simulink model "myBatteryValidationBlockDetailed2RC_IC"  (R2023a)
settings: Solver=daessc  StartTime=0.0  StopTime=1780.8908  MaxStep=1  RelTol=1e-3  AbsTol=1e-3
InitFcn:
  | batteryModelFromBlockDetailed2RC_IC_param
undefined symbols (not defined in the file or in its folder): battery_builder_rtmsupport, gcbh
libraries: batteryModelFromBlockDetailed2RC_IC_lib x36, fl_lib x3, nesl_utility x3
(part 2 of 3)

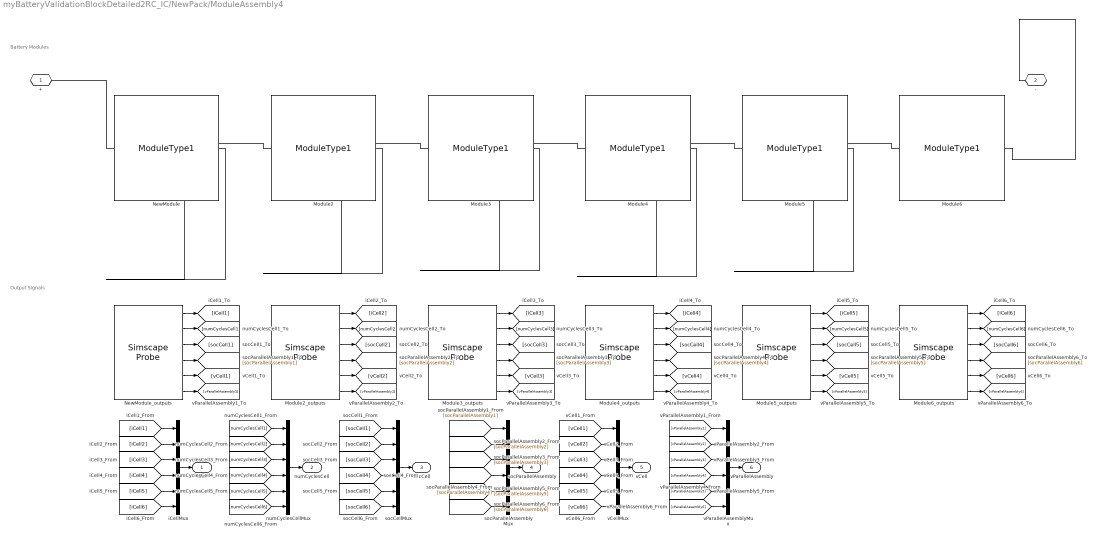
== system myBatteryValidationBlockDetailed2RC_IC/NewPack/ModuleAssembly4 ==
  note: Output Signals
  note: Battery Modules
  Module2 : batteryModelFromBlockDetailed2RC_IC_lib/Modules/ModuleType1  SOC_vecCell=ModuleType1.SOC_vecCell  V0_vecCell=ModuleType1.V0_vecCell V  V_rangeCell=ModuleType1.V_rangeCell V  R0_vecCell=ModuleType1.R0_vecCell Ohm  AHCell=ModuleType1.AHCell A*hr  extrapolation_optionCell=simscape.enum.extrapolation.nearest  R1_vecCell=ModuleType1.R1_vecCell Ohm  tau1_vecCell=ModuleType1.tau1_vecCell s  R2_vecCell=ModuleType1.R2_vecCell Ohm  tau2_vecCell=ModuleType1.tau2_vecCell s  P=1  S=1  iCell_specify=on  iCell_priority=None  iCell=ModuleAssembly4.Module2.iCell A  iCell_nominal_specify=off  iCell_nominal_unit=A  iCell_nominal_value=1  vCell_specify=on  vCell_priority=None  vCell=ModuleAssembly4.Module2.vCell V  vCell_nominal_specify=off  vCell_nominal_unit=V  vCell_nominal_value=1  socCell_specify=on  socCell_priority=High  socCell=ModuleAssembly4.Module2.socCell  socCell_nominal_specify=off  socCell_nominal_unit=1  socCell_nominal_value=1  numCyclesCell_specify=on  numCyclesCell_priority=High  numCyclesCell=ModuleAssembly4.Module2.numCyclesCell  numCyclesCell_nominal_specify=off  numCyclesCell_nominal_unit=1  numCyclesCell_nominal_value=1  vParallelAssembly_specify=on  vParallelAssembly_priority=None  vParallelAssembly=ModuleAssembly4.Module2.vParallelAssembly V  vParallelAssembly_nominal_specify=off  vParallelAssembly_nominal_unit=V  vParallelAssembly_nominal_value=1  socParallelAssembly_specify=on  socParallelAssembly_priority=None  socParallelAssembly=ModuleAssembly4.Module2.socParallelAssembly  socParallelAssembly_nominal_specify=off  socParallelAssembly_nominal_unit=1  socParallelAssembly_nominal_value=1
      settings: InternalSimscapePortConfiguration="{\"Bottom\":[{\"id\":\"n\",\"label\":\"-\",\"type\":\"foundation.electrical.electrical\"}],\"Left\":[],\"Right\":[],\"Top\":[{\"id\":\"p\",\"label\":\"+\",\"type\":\"foundation.electrical.electrical\"}]}"
  Module2_outputs : SimscapeProbe  BoundBlock=3097  Variables={iCell, numCyclesCell, socCell, socParallelAssembly, vCell, vParallelAssembly}
  Module3 : batteryModelFromBlockDetailed2RC_IC_lib/Modules/ModuleType1  SOC_vecCell=ModuleType1.SOC_vecCell  V0_vecCell=ModuleType1.V0_vecCell V  V_rangeCell=ModuleType1.V_rangeCell V  R0_vecCell=ModuleType1.R0_vecCell Ohm  AHCell=ModuleType1.AHCell A*hr  extrapolation_optionCell=simscape.enum.extrapolation.nearest  R1_vecCell=ModuleType1.R1_vecCell Ohm  tau1_vecCell=ModuleType1.tau1_vecCell s  R2_vecCell=ModuleType1.R2_vecCell Ohm  tau2_vecCell=ModuleType1.tau2_vecCell s  P=1  S=1  iCell_specify=on  iCell_priority=None  iCell=ModuleAssembly4.Module3.iCell A  iCell_nominal_specify=off  iCell_nominal_unit=A  iCell_nominal_value=1  vCell_specify=on  vCell_priority=None  vCell=ModuleAssembly4.Module3.vCell V  vCell_nominal_specify=off  vCell_nominal_unit=V  vCell_nominal_value=1  socCell_specify=on  socCell_priority=High  socCell=ModuleAssembly4.Module3.socCell  socCell_nominal_specify=off  socCell_nominal_unit=1  socCell_nominal_value=1  numCyclesCell_specify=on  numCyclesCell_priority=High  numCyclesCell=ModuleAssembly4.Module3.numCyclesCell  numCyclesCell_nominal_specify=off  numCyclesCell_nominal_unit=1  numCyclesCell_nominal_value=1  vParallelAssembly_specify=on  vParallelAssembly_priority=None  vParallelAssembly=ModuleAssembly4.Module3.vParallelAssembly V  vParallelAssembly_nominal_specify=off  vParallelAssembly_nominal_unit=V  vParallelAssembly_nominal_value=1  socParallelAssembly_specify=on  socParallelAssembly_priority=None  socParallelAssembly=ModuleAssembly4.Module3.socParallelAssembly  socParallelAssembly_nominal_specify=off  socParallelAssembly_nominal_unit=1  socParallelAssembly_nominal_value=1
      settings: InternalSimscapePortConfiguration="{\"Bottom\":[{\"id\":\"n\",\"label\":\"-\",\"type\":\"foundation.electrical.electrical\"}],\"Left\":[],\"Right\":[],\"Top\":[{\"id\":\"p\",\"label\":\"+\",\"type\":\"foundation.electrical.electrical\"}]}"
  Module3_outputs : SimscapeProbe  BoundBlock=3099  Variables={iCell, numCyclesCell, socCell, socParallelAssembly, vCell, vParallelAssembly}
  Module4 : batteryModelFromBlockDetailed2RC_IC_lib/Modules/ModuleType1  SOC_vecCell=ModuleType1.SOC_vecCell  V0_vecCell=ModuleType1.V0_vecCell V  V_rangeCell=ModuleType1.V_rangeCell V  R0_vecCell=ModuleType1.R0_vecCell Ohm  AHCell=ModuleType1.AHCell A*hr  extrapolation_optionCell=simscape.enum.extrapolation.nearest  R1_vecCell=ModuleType1.R1_vecCell Ohm  tau1_vecCell=ModuleType1.tau1_vecCell s  R2_vecCell=ModuleType1.R2_vecCell Ohm  tau2_vecCell=ModuleType1.tau2_vecCell s  P=1  S=1  iCell_specify=on  iCell_priority=None  iCell=ModuleAssembly4.Module4.iCell A  iCell_nominal_specify=off  iCell_nominal_unit=A  iCell_nominal_value=1  vCell_specify=on  vCell_priority=None  vCell=ModuleAssembly4.Module4.vCell V  vCell_nominal_specify=off  vCell_nominal_unit=V  vCell_nominal_value=1  socCell_specify=on  socCell_priority=High  socCell=ModuleAssembly4.Module4.socCell  socCell_nominal_specify=off  socCell_nominal_unit=1  socCell_nominal_value=1  numCyclesCell_specify=on  numCyclesCell_priority=High  numCyclesCell=ModuleAssembly4.Module4.numCyclesCell  numCyclesCell_nominal_specify=off  numCyclesCell_nominal_unit=1  numCyclesCell_nominal_value=1  vParallelAssembly_specify=on  vParallelAssembly_priority=None  vParallelAssembly=ModuleAssembly4.Module4.vParallelAssembly V  vParallelAssembly_nominal_specify=off  vParallelAssembly_nominal_unit=V  vParallelAssembly_nominal_value=1  socParallelAssembly_specify=on  socParallelAssembly_priority=None  socParallelAssembly=ModuleAssembly4.Module4.socParallelAssembly  socParallelAssembly_nominal_specify=off  socParallelAssembly_nominal_unit=1  socParallelAssembly_nominal_value=1
      settings: InternalSimscapePortConfiguration="{\"Bottom\":[{\"id\":\"n\",\"label\":\"-\",\"type\":\"foundation.electrical.electrical\"}],\"Left\":[],\"Right\":[],\"Top\":[{\"id\":\"p\",\"label\":\"+\",\"type\":\"foundation.electrical.electrical\"}]}"
  Module4_outputs : SimscapeProbe  BoundBlock=3101  Variables={iCell, numCyclesCell, socCell, socParallelAssembly, vCell, vParallelAssembly}
  Module5 : batteryModelFromBlockDetailed2RC_IC_lib/Modules/ModuleType1  SOC_vecCell=ModuleType1.SOC_vecCell  V0_vecCell=ModuleType1.V0_vecCell V  V_rangeCell=ModuleType1.V_rangeCell V  R0_vecCell=ModuleType1.R0_vecCell Ohm  AHCell=ModuleType1.AHCell A*hr  extrapolation_optionCell=simscape.enum.extrapolation.nearest  R1_vecCell=ModuleType1.R1_vecCell Ohm  tau1_vecCell=ModuleType1.tau1_vecCell s  R2_vecCell=ModuleType1.R2_vecCell Ohm  tau2_vecCell=ModuleType1.tau2_vecCell s  P=1  S=1  iCell_specify=on  iCell_priority=None  iCell=ModuleAssembly4.Module5.iCell A  iCell_nominal_specify=off  iCell_nominal_unit=A  iCell_nominal_value=1  vCell_specify=on  vCell_priority=None  vCell=ModuleAssembly4.Module5.vCell V  vCell_nominal_specify=off  vCell_nominal_unit=V  vCell_nominal_value=1  socCell_specify=on  socCell_priority=High  socCell=ModuleAssembly4.Module5.socCell  socCell_nominal_specify=off  socCell_nominal_unit=1  socCell_nominal_value=1  numCyclesCell_specify=on  numCyclesCell_priority=High  numCyclesCell=ModuleAssembly4.Module5.numCyclesCell  numCyclesCell_nominal_specify=off  numCyclesCell_nominal_unit=1  numCyclesCell_nominal_value=1  vParallelAssembly_specify=on  vParallelAssembly_priority=None  vParallelAssembly=ModuleAssembly4.Module5.vParallelAssembly V  vParallelAssembly_nominal_specify=off  vParallelAssembly_nominal_unit=V  vParallelAssembly_nominal_value=1  socParallelAssembly_specify=on  socParallelAssembly_priority=None  socParallelAssembly=ModuleAssembly4.Module5.socParallelAssembly  socParallelAssembly_nominal_specify=off  socParallelAssembly_nominal_unit=1  socParallelAssembly_nominal_value=1
      settings: InternalSimscapePortConfiguration="{\"Bottom\":[{\"id\":\"n\",\"label\":\"-\",\"type\":\"foundation.electrical.electrical\"}],\"Left\":[],\"Right\":[],\"Top\":[{\"id\":\"p\",\"label\":\"+\",\"type\":\"foundation.electrical.electrical\"}]}"
  Module5_outputs : SimscapeProbe  BoundBlock=3103  Variables={iCell, numCyclesCell, socCell, socParallelAssembly, vCell, vParallelAssembly}
  Module6 : batteryModelFromBlockDetailed2RC_IC_lib/Modules/ModuleType1  SOC_vecCell=ModuleType1.SOC_vecCell  V0_vecCell=ModuleType1.V0_vecCell V  V_rangeCell=ModuleType1.V_rangeCell V  R0_vecCell=ModuleType1.R0_vecCell Ohm  AHCell=ModuleType1.AHCell A*hr  extrapolation_optionCell=simscape.enum.extrapolation.nearest  R1_vecCell=ModuleType1.R1_vecCell Ohm  tau1_vecCell=ModuleType1.tau1_vecCell s  R2_vecCell=ModuleType1.R2_vecCell Ohm  tau2_vecCell=ModuleType1.tau2_vecCell s  P=1  S=1  iCell_specify=on  iCell_priority=None  iCell=ModuleAssembly4.Module6.iCell A  iCell_nominal_specify=off  iCell_nominal_unit=A  iCell_nominal_value=1  vCell_specify=on  vCell_priority=None  vCell=ModuleAssembly4.Module6.vCell V  vCell_nominal_specify=off  vCell_nominal_unit=V  vCell_nominal_value=1  socCell_specify=on  socCell_priority=High  socCell=ModuleAssembly4.Module6.socCell  socCell_nominal_specify=off  socCell_nominal_unit=1  socCell_nominal_value=1  numCyclesCell_specify=on  numCyclesCell_priority=High  numCyclesCell=ModuleAssembly4.Module6.numCyclesCell  numCyclesCell_nominal_specify=off  numCyclesCell_nominal_unit=1  numCyclesCell_nominal_value=1  vParallelAssembly_specify=on  vParallelAssembly_priority=None  vParallelAssembly=ModuleAssembly4.Module6.vParallelAssembly V  vParallelAssembly_nominal_specify=off  vParallelAssembly_nominal_unit=V  vParallelAssembly_nominal_value=1  socParallelAssembly_specify=on  socParallelAssembly_priority=None  socParallelAssembly=ModuleAssembly4.Module6.socParallelAssembly  socParallelAssembly_nominal_specify=off  socParallelAssembly_nominal_unit=1  socParallelAssembly_nominal_value=1
      settings: InternalSimscapePortConfiguration="{\"Bottom\":[{\"id\":\"n\",\"label\":\"-\",\"type\":\"foundation.electrical.electrical\"}],\"Left\":[],\"Right\":[],\"Top\":[{\"id\":\"p\",\"label\":\"+\",\"type\":\"foundation.electrical.electrical\"}]}"
  Module6_outputs : SimscapeProbe  BoundBlock=3105  Variables={iCell, numCyclesCell, socCell, socParallelAssembly, vCell, vParallelAssembly}
  NewModule : batteryModelFromBlockDetailed2RC_IC_lib/Modules/ModuleType1  SOC_vecCell=ModuleType1.SOC_vecCell  V0_vecCell=ModuleType1.V0_vecCell V  V_rangeCell=ModuleType1.V_rangeCell V  R0_vecCell=ModuleType1.R0_vecCell Ohm  AHCell=ModuleType1.AHCell A*hr  extrapolation_optionCell=simscape.enum.extrapolation.nearest  R1_vecCell=ModuleType1.R1_vecCell Ohm  tau1_vecCell=ModuleType1.tau1_vecCell s  R2_vecCell=ModuleType1.R2_vecCell Ohm  tau2_vecCell=ModuleType1.tau2_vecCell s  P=1  S=1  iCell_specify=on  iCell_priority=None  iCell=ModuleAssembly4.NewModule.iCell A  iCell_nominal_specify=off  iCell_nominal_unit=A  iCell_nominal_value=1  vCell_specify=on  vCell_priority=None  vCell=ModuleAssembly4.NewModule.vCell V  vCell_nominal_specify=off  vCell_nominal_unit=V  vCell_nominal_value=1  socCell_specify=on  socCell_priority=High  socCell=ModuleAssembly4.NewModule.socCell  socCell_nominal_specify=off  socCell_nominal_unit=1  socCell_nominal_value=1  numCyclesCell_specify=on  numCyclesCell_priority=High  numCyclesCell=ModuleAssembly4.NewModule.numCyclesCell  numCyclesCell_nominal_specify=off  numCyclesCell_nominal_unit=1  numCyclesCell_nominal_value=1  vParallelAssembly_specify=on  vParallelAssembly_priority=None  vParallelAssembly=ModuleAssembly4.NewModule.vParallelAssembly V  vParallelAssembly_nominal_specify=off  vParallelAssembly_nominal_unit=V  vParallelAssembly_nominal_value=1  socParallelAssembly_specify=on  socParallelAssembly_priority=None  socParallelAssembly=ModuleAssembly4.NewModule.socParallelAssembly  socParallelAssembly_nominal_specify=off  socParallelAssembly_nominal_unit=1  socParallelAssembly_nominal_value=1
      settings: InternalSimscapePortConfiguration="{\"Bottom\":[{\"id\":\"n\",\"label\":\"-\",\"type\":\"foundation.electrical.electrical\"}],\"Left\":[],\"Right\":[],\"Top\":[{\"id\":\"p\",\"label\":\"+\",\"type\":\"foundation.electrical.electrical\"}]}"
  NewModule_outputs : SimscapeProbe  BoundBlock=3107  Variables={iCell, numCyclesCell, socCell, socParallelAssembly, vCell, vParallelAssembly}
  iCellMux : Mux  Inputs=6
  numCyclesCellMux : Mux  Inputs=6
  socCellMux : Mux  Inputs=6
  socParallelAssemblyMux : Mux  Inputs=6
  vCellMux : Mux  Inputs=6
  vParallelAssemblyMux : Mux  Inputs=6
  + : PMIOPort  Side=Left
  - : PMIOPort  Port=2  Side=Right
  iCell : Outport
  numCyclesCell : Outport  Port=2
  socCell : Outport  Port=3
  socParallelAssembly : Outport  Port=4
  vCell : Outport  Port=5
  vParallelAssembly : Outport  Port=6
  wires:
  [vParallelAssembly6] -> vParallelAssemblyMux/6
  Module6_outputs/6 -> [vParallelAssembly6]
  [vCell6] -> vCellMux/6
  Module6_outputs/5 -> [vCell6]
  [socParallelAssembly6] -> socParallelAssemblyMux/6
  Module6_outputs/4 -> [socParallelAssembly6]
  [socCell6] -> socCellMux/6
  Module6_outputs/3 -> [socCell6]
  [numCyclesCell6] -> numCyclesCellMux/6
  Module6_outputs/2 -> [numCyclesCell6]
  [iCell6] -> iCellMux/6
  Module6_outputs/1 -> [iCell6]
  [vParallelAssembly5] -> vParallelAssemblyMux/5
  Module5_outputs/6 -> [vParallelAssembly5]
  [vCell5] -> vCellMux/5
  Module5_outputs/5 -> [vCell5]
  [socParallelAssembly5] -> socParallelAssemblyMux/5
  Module5_outputs/4 -> [socParallelAssembly5]
  [socCell5] -> socCellMux/5
  Module5_outputs/3 -> [socCell5]
  [numCyclesCell5] -> numCyclesCellMux/5
  Module5_outputs/2 -> [numCyclesCell5]
  [iCell5] -> iCellMux/5
  Module5_outputs/1 -> [iCell5]
  [vParallelAssembly4] -> vParallelAssemblyMux/4
  Module4_outputs/6 -> [vParallelAssembly4]
  [vCell4] -> vCellMux/4
  Module4_outputs/5 -> [vCell4]
  [socParallelAssembly4] -> socParallelAssemblyMux/4
  Module4_outputs/4 -> [socParallelAssembly4]
  [socCell4] -> socCellMux/4
  Module4_outputs/3 -> [socCell4]
  [numCyclesCell4] -> numCyclesCellMux/4
  Module4_outputs/2 -> [numCyclesCell4]
  [iCell4] -> iCellMux/4
  Module4_outputs/1 -> [iCell4]
  [vParallelAssembly3] -> vParallelAssemblyMux/3
  Module3_outputs/6 -> [vParallelAssembly3]
  [vCell3] -> vCellMux/3
  Module3_outputs/5 -> [vCell3]
  [socParallelAssembly3] -> socParallelAssemblyMux/3
  Module3_outputs/4 -> [socParallelAssembly3]
  [socCell3] -> socCellMux/3
  Module3_outputs/3 -> [socCell3]
  [numCyclesCell3] -> numCyclesCellMux/3
  Module3_outputs/2 -> [numCyclesCell3]
  [iCell3] -> iCellMux/3
  Module3_outputs/1 -> [iCell3]
  [vParallelAssembly2] -> vParallelAssemblyMux/2
  Module2_outputs/6 -> [vParallelAssembly2]
  [vCell2] -> vCellMux/2
  Module2_outputs/5 -> [vCell2]
  [socParallelAssembly2] -> socParallelAssemblyMux/2
  Module2_outputs/4 -> [socParallelAssembly2]
  [socCell2] -> socCellMux/2
  Module2_outputs/3 -> [socCell2]
  [numCyclesCell2] -> numCyclesCellMux/2
  Module2_outputs/2 -> [numCyclesCell2]
  [iCell2] -> iCellMux/2
  Module2_outputs/1 -> [iCell2]
  [vParallelAssembly1] -> vParallelAssemblyMux/1
  vParallelAssemblyMux/1 -> vParallelAssembly/1
  NewModule_outputs/6 -> [vParallelAssembly1]
  [vCell1] -> vCellMux/1
  vCellMux/1 -> vCell/1
  NewModule_outputs/5 -> [vCell1]
  [socParallelAssembly1] -> socParallelAssemblyMux/1
  socParallelAssemblyMux/1 -> socParallelAssembly/1
  NewModule_outputs/4 -> [socParallelAssembly1]
  [socCell1] -> socCellMux/1
  socCellMux/1 -> socCell/1
  NewModule_outputs/3 -> [socCell1]
  [numCyclesCell1] -> numCyclesCellMux/1
  numCyclesCellMux/1 -> numCyclesCell/1
  NewModule_outputs/2 -> [numCyclesCell1]
  [iCell1] -> iCellMux/1
  iCellMux/1 -> iCell/1
  NewModule_outputs/1 -> [iCell1]
  connections:
  Module6/RConn1 -- -/RConn1
  NewModule/LConn1 -- +/RConn1
  Module6/LConn1 -- Module5/RConn1
  Module5/LConn1 -- Module4/RConn1
  Module4/LConn1 -- Module3/RConn1
  Module3/LConn1 -- Module2/RConn1
  Module2/LConn1 -- NewModule/RConn1

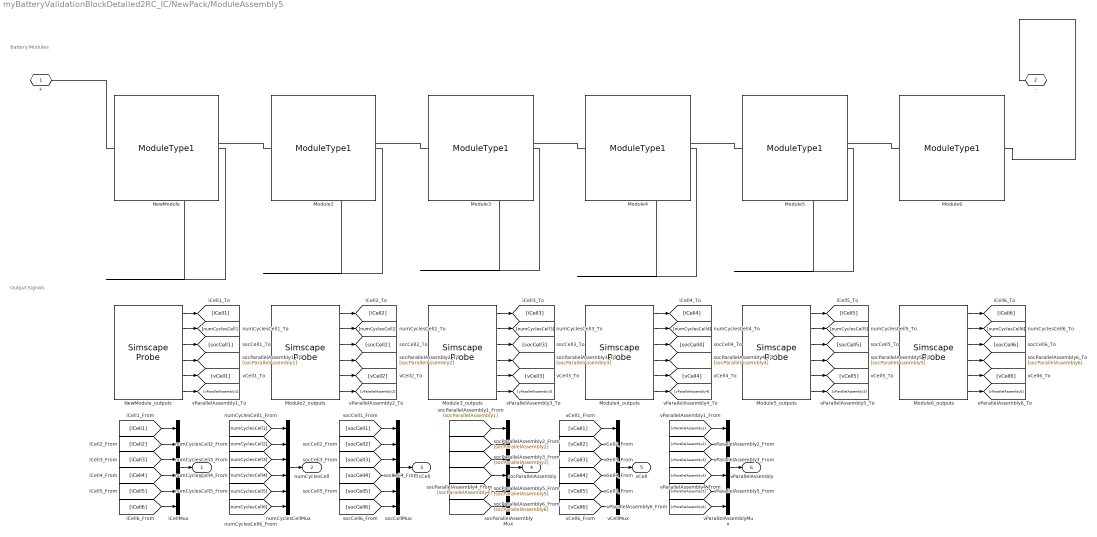
== system myBatteryValidationBlockDetailed2RC_IC/NewPack/ModuleAssembly5 ==
  note: Output Signals
  note: Battery Modules
  Module2 : batteryModelFromBlockDetailed2RC_IC_lib/Modules/ModuleType1  SOC_vecCell=ModuleType1.SOC_vecCell  V0_vecCell=ModuleType1.V0_vecCell V  V_rangeCell=ModuleType1.V_rangeCell V  R0_vecCell=ModuleType1.R0_vecCell Ohm  AHCell=ModuleType1.AHCell A*hr  extrapolation_optionCell=simscape.enum.extrapolation.nearest  R1_vecCell=ModuleType1.R1_vecCell Ohm  tau1_vecCell=ModuleType1.tau1_vecCell s  R2_vecCell=ModuleType1.R2_vecCell Ohm  tau2_vecCell=ModuleType1.tau2_vecCell s  P=1  S=1  iCell_specify=on  iCell_priority=None  iCell=ModuleAssembly5.Module2.iCell A  iCell_nominal_specify=off  iCell_nominal_unit=A  iCell_nominal_value=1  vCell_specify=on  vCell_priority=None  vCell=ModuleAssembly5.Module2.vCell V  vCell_nominal_specify=off  vCell_nominal_unit=V  vCell_nominal_value=1  socCell_specify=on  socCell_priority=High  socCell=ModuleAssembly5.Module2.socCell  socCell_nominal_specify=off  socCell_nominal_unit=1  socCell_nominal_value=1  numCyclesCell_specify=on  numCyclesCell_priority=High  numCyclesCell=ModuleAssembly5.Module2.numCyclesCell  numCyclesCell_nominal_specify=off  numCyclesCell_nominal_unit=1  numCyclesCell_nominal_value=1  vParallelAssembly_specify=on  vParallelAssembly_priority=None  vParallelAssembly=ModuleAssembly5.Module2.vParallelAssembly V  vParallelAssembly_nominal_specify=off  vParallelAssembly_nominal_unit=V  vParallelAssembly_nominal_value=1  socParallelAssembly_specify=on  socParallelAssembly_priority=None  socParallelAssembly=ModuleAssembly5.Module2.socParallelAssembly  socParallelAssembly_nominal_specify=off  socParallelAssembly_nominal_unit=1  socParallelAssembly_nominal_value=1
      settings: InternalSimscapePortConfiguration="{\"Bottom\":[{\"id\":\"n\",\"label\":\"-\",\"type\":\"foundation.electrical.electrical\"}],\"Left\":[],\"Right\":[],\"Top\":[{\"id\":\"p\",\"label\":\"+\",\"type\":\"foundation.electrical.electrical\"}]}"
  Module2_outputs : SimscapeProbe  BoundBlock=3198  Variables={iCell, numCyclesCell, socCell, socParallelAssembly, vCell, vParallelAssembly}
  Module3 : batteryModelFromBlockDetailed2RC_IC_lib/Modules/ModuleType1  SOC_vecCell=ModuleType1.SOC_vecCell  V0_vecCell=ModuleType1.V0_vecCell V  V_rangeCell=ModuleType1.V_rangeCell V  R0_vecCell=ModuleType1.R0_vecCell Ohm  AHCell=ModuleType1.AHCell A*hr  extrapolation_optionCell=simscape.enum.extrapolation.nearest  R1_vecCell=ModuleType1.R1_vecCell Ohm  tau1_vecCell=ModuleType1.tau1_vecCell s  R2_vecCell=ModuleType1.R2_vecCell Ohm  tau2_vecCell=ModuleType1.tau2_vecCell s  P=1  S=1  iCell_specify=on  iCell_priority=None  iCell=ModuleAssembly5.Module3.iCell A  iCell_nominal_specify=off  iCell_nominal_unit=A  iCell_nominal_value=1  vCell_specify=on  vCell_priority=None  vCell=ModuleAssembly5.Module3.vCell V  vCell_nominal_specify=off  vCell_nominal_unit=V  vCell_nominal_value=1  socCell_specify=on  socCell_priority=High  socCell=ModuleAssembly5.Module3.socCell  socCell_nominal_specify=off  socCell_nominal_unit=1  socCell_nominal_value=1  numCyclesCell_specify=on  numCyclesCell_priority=High  numCyclesCell=ModuleAssembly5.Module3.numCyclesCell  numCyclesCell_nominal_specify=off  numCyclesCell_nominal_unit=1  numCyclesCell_nominal_value=1  vParallelAssembly_specify=on  vParallelAssembly_priority=None  vParallelAssembly=ModuleAssembly5.Module3.vParallelAssembly V  vParallelAssembly_nominal_specify=off  vParallelAssembly_nominal_unit=V  vParallelAssembly_nominal_value=1  socParallelAssembly_specify=on  socParallelAssembly_priority=None  socParallelAssembly=ModuleAssembly5.Module3.socParallelAssembly  socParallelAssembly_nominal_specify=off  socParallelAssembly_nominal_unit=1  socParallelAssembly_nominal_value=1
      settings: InternalSimscapePortConfiguration="{\"Bottom\":[{\"id\":\"n\",\"label\":\"-\",\"type\":\"foundation.electrical.electrical\"}],\"Left\":[],\"Right\":[],\"Top\":[{\"id\":\"p\",\"label\":\"+\",\"type\":\"foundation.electrical.electrical\"}]}"
  Module3_outputs : SimscapeProbe  BoundBlock=3200  Variables={iCell, numCyclesCell, socCell, socParallelAssembly, vCell, vParallelAssembly}
  Module4 : batteryModelFromBlockDetailed2RC_IC_lib/Modules/ModuleType1  SOC_vecCell=ModuleType1.SOC_vecCell  V0_vecCell=ModuleType1.V0_vecCell V  V_rangeCell=ModuleType1.V_rangeCell V  R0_vecCell=ModuleType1.R0_vecCell Ohm  AHCell=ModuleType1.AHCell A*hr  extrapolation_optionCell=simscape.enum.extrapolation.nearest  R1_vecCell=ModuleType1.R1_vecCell Ohm  tau1_vecCell=ModuleType1.tau1_vecCell s  R2_vecCell=ModuleType1.R2_vecCell Ohm  tau2_vecCell=ModuleType1.tau2_vecCell s  P=1  S=1  iCell_specify=on  iCell_priority=None  iCell=ModuleAssembly5.Module4.iCell A  iCell_nominal_specify=off  iCell_nominal_unit=A  iCell_nominal_value=1  vCell_specify=on  vCell_priority=None  vCell=ModuleAssembly5.Module4.vCell V  vCell_nominal_specify=off  vCell_nominal_unit=V  vCell_nominal_value=1  socCell_specify=on  socCell_priority=High  socCell=ModuleAssembly5.Module4.socCell  socCell_nominal_specify=off  socCell_nominal_unit=1  socCell_nominal_value=1  numCyclesCell_specify=on  numCyclesCell_priority=High  numCyclesCell=ModuleAssembly5.Module4.numCyclesCell  numCyclesCell_nominal_specify=off  numCyclesCell_nominal_unit=1  numCyclesCell_nominal_value=1  vParallelAssembly_specify=on  vParallelAssembly_priority=None  vParallelAssembly=ModuleAssembly5.Module4.vParallelAssembly V  vParallelAssembly_nominal_specify=off  vParallelAssembly_nominal_unit=V  vParallelAssembly_nominal_value=1  socParallelAssembly_specify=on  socParallelAssembly_priority=None  socParallelAssembly=ModuleAssembly5.Module4.socParallelAssembly  socParallelAssembly_nominal_specify=off  socParallelAssembly_nominal_unit=1  socParallelAssembly_nominal_value=1
      settings: InternalSimscapePortConfiguration="{\"Bottom\":[{\"id\":\"n\",\"label\":\"-\",\"type\":\"foundation.electrical.electrical\"}],\"Left\":[],\"Right\":[],\"Top\":[{\"id\":\"p\",\"label\":\"+\",\"type\":\"foundation.electrical.electrical\"}]}"
  Module4_outputs : SimscapeProbe  BoundBlock=3202  Variables={iCell, numCyclesCell, socCell, socParallelAssembly, vCell, vParallelAssembly}
  Module5 : batteryModelFromBlockDetailed2RC_IC_lib/Modules/ModuleType1  SOC_vecCell=ModuleType1.SOC_vecCell  V0_vecCell=ModuleType1.V0_vecCell V  V_rangeCell=ModuleType1.V_rangeCell V  R0_vecCell=ModuleType1.R0_vecCell Ohm  AHCell=ModuleType1.AHCell A*hr  extrapolation_optionCell=simscape.enum.extrapolation.nearest  R1_vecCell=ModuleType1.R1_vecCell Ohm  tau1_vecCell=ModuleType1.tau1_vecCell s  R2_vecCell=ModuleType1.R2_vecCell Ohm  tau2_vecCell=ModuleType1.tau2_vecCell s  P=1  S=1  iCell_specify=on  iCell_priority=None  iCell=ModuleAssembly5.Module5.iCell A  iCell_nominal_specify=off  iCell_nominal_unit=A  iCell_nominal_value=1  vCell_specify=on  vCell_priority=None  vCell=ModuleAssembly5.Module5.vCell V  vCell_nominal_specify=off  vCell_nominal_unit=V  vCell_nominal_value=1  socCell_specify=on  socCell_priority=High  socCell=ModuleAssembly5.Module5.socCell  socCell_nominal_specify=off  socCell_nominal_unit=1  socCell_nominal_value=1  numCyclesCell_specify=on  numCyclesCell_priority=High  numCyclesCell=ModuleAssembly5.Module5.numCyclesCell  numCyclesCell_nominal_specify=off  numCyclesCell_nominal_unit=1  numCyclesCell_nominal_value=1  vParallelAssembly_specify=on  vParallelAssembly_priority=None  vParallelAssembly=ModuleAssembly5.Module5.vParallelAssembly V  vParallelAssembly_nominal_specify=off  vParallelAssembly_nominal_unit=V  vParallelAssembly_nominal_value=1  socParallelAssembly_specify=on  socParallelAssembly_priority=None  socParallelAssembly=ModuleAssembly5.Module5.socParallelAssembly  socParallelAssembly_nominal_specify=off  socParallelAssembly_nominal_unit=1  socParallelAssembly_nominal_value=1
      settings: InternalSimscapePortConfiguration="{\"Bottom\":[{\"id\":\"n\",\"label\":\"-\",\"type\":\"foundation.electrical.electrical\"}],\"Left\":[],\"Right\":[],\"Top\":[{\"id\":\"p\",\"label\":\"+\",\"type\":\"foundation.electrical.electrical\"}]}"
  Module5_outputs : SimscapeProbe  BoundBlock=3204  Variables={iCell, numCyclesCell, socCell, socParallelAssembly, vCell, vParallelAssembly}
  Module6 : batteryModelFromBlockDetailed2RC_IC_lib/Modules/ModuleType1  SOC_vecCell=ModuleType1.SOC_vecCell  V0_vecCell=ModuleType1.V0_vecCell V  V_rangeCell=ModuleType1.V_rangeCell V  R0_vecCell=ModuleType1.R0_vecCell Ohm  AHCell=ModuleType1.AHCell A*hr  extrapolation_optionCell=simscape.enum.extrapolation.nearest  R1_vecCell=ModuleType1.R1_vecCell Ohm  tau1_vecCell=ModuleType1.tau1_vecCell s  R2_vecCell=ModuleType1.R2_vecCell Ohm  tau2_vecCell=ModuleType1.tau2_vecCell s  P=1  S=1  iCell_specify=on  iCell_priority=None  iCell=ModuleAssembly5.Module6.iCell A  iCell_nominal_specify=off  iCell_nominal_unit=A  iCell_nominal_value=1  vCell_specify=on  vCell_priority=None  vCell=ModuleAssembly5.Module6.vCell V  vCell_nominal_specify=off  vCell_nominal_unit=V  vCell_nominal_value=1  socCell_specify=on  socCell_priority=High  socCell=ModuleAssembly5.Module6.socCell  socCell_nominal_specify=off  socCell_nominal_unit=1  socCell_nominal_value=1  numCyclesCell_specify=on  numCyclesCell_priority=High  numCyclesCell=ModuleAssembly5.Module6.numCyclesCell  numCyclesCell_nominal_specify=off  numCyclesCell_nominal_unit=1  numCyclesCell_nominal_value=1  vParallelAssembly_specify=on  vParallelAssembly_priority=None  vParallelAssembly=ModuleAssembly5.Module6.vParallelAssembly V  vParallelAssembly_nominal_specify=off  vParallelAssembly_nominal_unit=V  vParallelAssembly_nominal_value=1  socParallelAssembly_specify=on  socParallelAssembly_priority=None  socParallelAssembly=ModuleAssembly5.Module6.socParallelAssembly  socParallelAssembly_nominal_specify=off  socParallelAssembly_nominal_unit=1  socParallelAssembly_nominal_value=1
      settings: InternalSimscapePortConfiguration="{\"Bottom\":[{\"id\":\"n\",\"label\":\"-\",\"type\":\"foundation.electrical.electrical\"}],\"Left\":[],\"Right\":[],\"Top\":[{\"id\":\"p\",\"label\":\"+\",\"type\":\"foundation.electrical.electrical\"}]}"
  Module6_outputs : SimscapeProbe  BoundBlock=3206  Variables={iCell, numCyclesCell, socCell, socParallelAssembly, vCell, vParallelAssembly}
  NewModule : batteryModelFromBlockDetailed2RC_IC_lib/Modules/ModuleType1  SOC_vecCell=ModuleType1.SOC_vecCell  V0_vecCell=ModuleType1.V0_vecCell V  V_rangeCell=ModuleType1.V_rangeCell V  R0_vecCell=ModuleType1.R0_vecCell Ohm  AHCell=ModuleType1.AHCell A*hr  extrapolation_optionCell=simscape.enum.extrapolation.nearest  R1_vecCell=ModuleType1.R1_vecCell Ohm  tau1_vecCell=ModuleType1.tau1_vecCell s  R2_vecCell=ModuleType1.R2_vecCell Ohm  tau2_vecCell=ModuleType1.tau2_vecCell s  P=1  S=1  iCell_specify=on  iCell_priority=None  iCell=ModuleAssembly5.NewModule.iCell A  iCell_nominal_specify=off  iCell_nominal_unit=A  iCell_nominal_value=1  vCell_specify=on  vCell_priority=None  vCell=ModuleAssembly5.NewModule.vCell V  vCell_nominal_specify=off  vCell_nominal_unit=V  vCell_nominal_value=1  socCell_specify=on  socCell_priority=High  socCell=ModuleAssembly5.NewModule.socCell  socCell_nominal_specify=off  socCell_nominal_unit=1  socCell_nominal_value=1  numCyclesCell_specify=on  numCyclesCell_priority=High  numCyclesCell=ModuleAssembly5.NewModule.numCyclesCell  numCyclesCell_nominal_specify=off  numCyclesCell_nominal_unit=1  numCyclesCell_nominal_value=1  vParallelAssembly_specify=on  vParallelAssembly_priority=None  vParallelAssembly=ModuleAssembly5.NewModule.vParallelAssembly V  vParallelAssembly_nominal_specify=off  vParallelAssembly_nominal_unit=V  vParallelAssembly_nominal_value=1  socParallelAssembly_specify=on  socParallelAssembly_priority=None  socParallelAssembly=ModuleAssembly5.NewModule.socParallelAssembly  socParallelAssembly_nominal_specify=off  socParallelAssembly_nominal_unit=1  socParallelAssembly_nominal_value=1
      settings: InternalSimscapePortConfiguration="{\"Bottom\":[{\"id\":\"n\",\"label\":\"-\",\"type\":\"foundation.electrical.electrical\"}],\"Left\":[],\"Right\":[],\"Top\":[{\"id\":\"p\",\"label\":\"+\",\"type\":\"foundation.electrical.electrical\"}]}"
  NewModule_outputs : SimscapeProbe  BoundBlock=3208  Variables={iCell, numCyclesCell, socCell, socParallelAssembly, vCell, vParallelAssembly}
  iCellMux : Mux  Inputs=6
  numCyclesCellMux : Mux  Inputs=6
  socCellMux : Mux  Inputs=6
  socParallelAssemblyMux : Mux  Inputs=6
  vCellMux : Mux  Inputs=6
  vParallelAssemblyMux : Mux  Inputs=6
  + : PMIOPort  Side=Left
  - : PMIOPort  Port=2  Side=Right
  iCell : Outport
  numCyclesCell : Outport  Port=2
  socCell : Outport  Port=3
  socParallelAssembly : Outport  Port=4
  vCell : Outport  Port=5
  vParallelAssembly : Outport  Port=6
  wires:
  [vParallelAssembly6] -> vParallelAssemblyMux/6
  Module6_outputs/6 -> [vParallelAssembly6]
  [vCell6] -> vCellMux/6
  Module6_outputs/5 -> [vCell6]
  [socParallelAssembly6] -> socParallelAssemblyMux/6
  Module6_outputs/4 -> [socParallelAssembly6]
  [socCell6] -> socCellMux/6
  Module6_outputs/3 -> [socCell6]
  [numCyclesCell6] -> numCyclesCellMux/6
  Module6_outputs/2 -> [numCyclesCell6]
  [iCell6] -> iCellMux/6
  Module6_outputs/1 -> [iCell6]
  [vParallelAssembly5] -> vParallelAssemblyMux/5
  Module5_outputs/6 -> [vParallelAssembly5]
  [vCell5] -> vCellMux/5
  Module5_outputs/5 -> [vCell5]
  [socParallelAssembly5] -> socParallelAssemblyMux/5
  Module5_outputs/4 -> [socParallelAssembly5]
  [socCell5] -> socCellMux/5
  Module5_outputs/3 -> [socCell5]
  [numCyclesCell5] -> numCyclesCellMux/5
  Module5_outputs/2 -> [numCyclesCell5]
  [iCell5] -> iCellMux/5
  Module5_outputs/1 -> [iCell5]
  [vParallelAssembly4] -> vParallelAssemblyMux/4
  Module4_outputs/6 -> [vParallelAssembly4]
  [vCell4] -> vCellMux/4
  Module4_outputs/5 -> [vCell4]
  [socParallelAssembly4] -> socParallelAssemblyMux/4
  Module4_outputs/4 -> [socParallelAssembly4]
  [socCell4] -> socCellMux/4
  Module4_outputs/3 -> [socCell4]
  [numCyclesCell4] -> numCyclesCellMux/4
  Module4_outputs/2 -> [numCyclesCell4]
  [iCell4] -> iCellMux/4
  Module4_outputs/1 -> [iCell4]
  [vParallelAssembly3] -> vParallelAssemblyMux/3
  Module3_outputs/6 -> [vParallelAssembly3]
  [vCell3] -> vCellMux/3
  Module3_outputs/5 -> [vCell3]
  [socParallelAssembly3] -> socParallelAssemblyMux/3
  Module3_outputs/4 -> [socParallelAssembly3]
  [socCell3] -> socCellMux/3
  Module3_outputs/3 -> [socCell3]
  [numCyclesCell3] -> numCyclesCellMux/3
  Module3_outputs/2 -> [numCyclesCell3]
  [iCell3] -> iCellMux/3
  Module3_outputs/1 -> [iCell3]
  [vParallelAssembly2] -> vParallelAssemblyMux/2
  Module2_outputs/6 -> [vParallelAssembly2]
  [vCell2] -> vCellMux/2
  Module2_outputs/5 -> [vCell2]
  [socParallelAssembly2] -> socParallelAssemblyMux/2
  Module2_outputs/4 -> [socParallelAssembly2]
  [socCell2] -> socCellMux/2
  Module2_outputs/3 -> [socCell2]
  [numCyclesCell2] -> numCyclesCellMux/2
  Module2_outputs/2 -> [numCyclesCell2]
  [iCell2] -> iCellMux/2
  Module2_outputs/1 -> [iCell2]
  [vParallelAssembly1] -> vParallelAssemblyMux/1
  vParallelAssemblyMux/1 -> vParallelAssembly/1
  NewModule_outputs/6 -> [vParallelAssembly1]
  [vCell1] -> vCellMux/1
  vCellMux/1 -> vCell/1
  NewModule_outputs/5 -> [vCell1]
  [socParallelAssembly1] -> socParallelAssemblyMux/1
  socParallelAssemblyMux/1 -> socParallelAssembly/1
  NewModule_outputs/4 -> [socParallelAssembly1]
  [socCell1] -> socCellMux/1
  socCellMux/1 -> socCell/1
  NewModule_outputs/3 -> [socCell1]
  [numCyclesCell1] -> numCyclesCellMux/1
  numCyclesCellMux/1 -> numCyclesCell/1
  NewModule_outputs/2 -> [numCyclesCell1]
  [iCell1] -> iCellMux/1
  iCellMux/1 -> iCell/1
  NewModule_outputs/1 -> [iCell1]
  connections:
  Module6/RConn1 -- -/RConn1
  NewModule/LConn1 -- +/RConn1
  Module6/LConn1 -- Module5/RConn1
  Module5/LConn1 -- Module4/RConn1
  Module4/LConn1 -- Module3/RConn1
  Module3/LConn1 -- Module2/RConn1
  Module2/LConn1 -- NewModule/RConn1

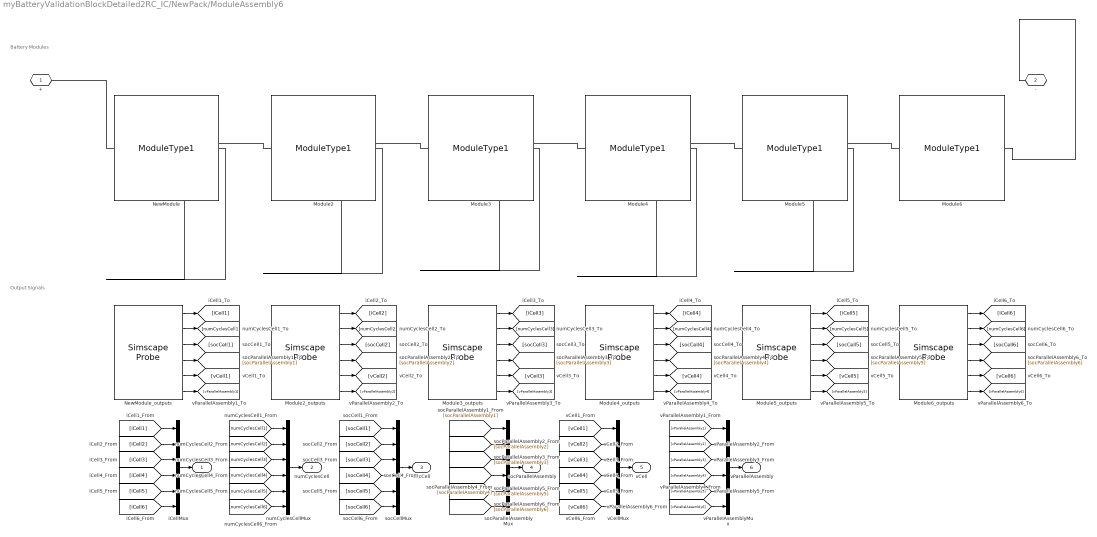
== system myBatteryValidationBlockDetailed2RC_IC/NewPack/ModuleAssembly6 ==
  note: Output Signals
  note: Battery Modules
  Module2 : batteryModelFromBlockDetailed2RC_IC_lib/Modules/ModuleType1  SOC_vecCell=ModuleType1.SOC_vecCell  V0_vecCell=ModuleType1.V0_vecCell V  V_rangeCell=ModuleType1.V_rangeCell V  R0_vecCell=ModuleType1.R0_vecCell Ohm  AHCell=ModuleType1.AHCell A*hr  extrapolation_optionCell=simscape.enum.extrapolation.nearest  R1_vecCell=ModuleType1.R1_vecCell Ohm  tau1_vecCell=ModuleType1.tau1_vecCell s  R2_vecCell=ModuleType1.R2_vecCell Ohm  tau2_vecCell=ModuleType1.tau2_vecCell s  P=1  S=1  iCell_specify=on  iCell_priority=None  iCell=ModuleAssembly6.Module2.iCell A  iCell_nominal_specify=off  iCell_nominal_unit=A  iCell_nominal_value=1  vCell_specify=on  vCell_priority=None  vCell=ModuleAssembly6.Module2.vCell V  vCell_nominal_specify=off  vCell_nominal_unit=V  vCell_nominal_value=1  socCell_specify=on  socCell_priority=High  socCell=ModuleAssembly6.Module2.socCell  socCell_nominal_specify=off  socCell_nominal_unit=1  socCell_nominal_value=1  numCyclesCell_specify=on  numCyclesCell_priority=High  numCyclesCell=ModuleAssembly6.Module2.numCyclesCell  numCyclesCell_nominal_specify=off  numCyclesCell_nominal_unit=1  numCyclesCell_nominal_value=1  vParallelAssembly_specify=on  vParallelAssembly_priority=None  vParallelAssembly=ModuleAssembly6.Module2.vParallelAssembly V  vParallelAssembly_nominal_specify=off  vParallelAssembly_nominal_unit=V  vParallelAssembly_nominal_value=1  socParallelAssembly_specify=on  socParallelAssembly_priority=None  socParallelAssembly=ModuleAssembly6.Module2.socParallelAssembly  socParallelAssembly_nominal_specify=off  socParallelAssembly_nominal_unit=1  socParallelAssembly_nominal_value=1
      settings: InternalSimscapePortConfiguration="{\"Bottom\":[{\"id\":\"n\",\"label\":\"-\",\"type\":\"foundation.electrical.electrical\"}],\"Left\":[],\"Right\":[],\"Top\":[{\"id\":\"p\",\"label\":\"+\",\"type\":\"foundation.electrical.electrical\"}]}"
  Module2_outputs : SimscapeProbe  BoundBlock=3299  Variables={iCell, numCyclesCell, socCell, socParallelAssembly, vCell, vParallelAssembly}
  Module3 : batteryModelFromBlockDetailed2RC_IC_lib/Modules/ModuleType1  SOC_vecCell=ModuleType1.SOC_vecCell  V0_vecCell=ModuleType1.V0_vecCell V  V_rangeCell=ModuleType1.V_rangeCell V  R0_vecCell=ModuleType1.R0_vecCell Ohm  AHCell=ModuleType1.AHCell A*hr  extrapolation_optionCell=simscape.enum.extrapolation.nearest  R1_vecCell=ModuleType1.R1_vecCell Ohm  tau1_vecCell=ModuleType1.tau1_vecCell s  R2_vecCell=ModuleType1.R2_vecCell Ohm  tau2_vecCell=ModuleType1.tau2_vecCell s  P=1  S=1  iCell_specify=on  iCell_priority=None  iCell=ModuleAssembly6.Module3.iCell A  iCell_nominal_specify=off  iCell_nominal_unit=A  iCell_nominal_value=1  vCell_specify=on  vCell_priority=None  vCell=ModuleAssembly6.Module3.vCell V  vCell_nominal_specify=off  vCell_nominal_unit=V  vCell_nominal_value=1  socCell_specify=on  socCell_priority=High  socCell=ModuleAssembly6.Module3.socCell  socCell_nominal_specify=off  socCell_nominal_unit=1  socCell_nominal_value=1  numCyclesCell_specify=on  numCyclesCell_priority=High  numCyclesCell=ModuleAssembly6.Module3.numCyclesCell  numCyclesCell_nominal_specify=off  numCyclesCell_nominal_unit=1  numCyclesCell_nominal_value=1  vParallelAssembly_specify=on  vParallelAssembly_priority=None  vParallelAssembly=ModuleAssembly6.Module3.vParallelAssembly V  vParallelAssembly_nominal_specify=off  vParallelAssembly_nominal_unit=V  vParallelAssembly_nominal_value=1  socParallelAssembly_specify=on  socParallelAssembly_priority=None  socParallelAssembly=ModuleAssembly6.Module3.socParallelAssembly  socParallelAssembly_nominal_specify=off  socParallelAssembly_nominal_unit=1  socParallelAssembly_nominal_value=1
      settings: InternalSimscapePortConfiguration="{\"Bottom\":[{\"id\":\"n\",\"label\":\"-\",\"type\":\"foundation.electrical.electrical\"}],\"Left\":[],\"Right\":[],\"Top\":[{\"id\":\"p\",\"label\":\"+\",\"type\":\"foundation.electrical.electrical\"}]}"
  Module3_outputs : SimscapeProbe  BoundBlock=3301  Variables={iCell, numCyclesCell, socCell, socParallelAssembly, vCell, vParallelAssembly}
  Module4 : batteryModelFromBlockDetailed2RC_IC_lib/Modules/ModuleType1  SOC_vecCell=ModuleType1.SOC_vecCell  V0_vecCell=ModuleType1.V0_vecCell V  V_rangeCell=ModuleType1.V_rangeCell V  R0_vecCell=ModuleType1.R0_vecCell Ohm  AHCell=ModuleType1.AHCell A*hr  extrapolation_optionCell=simscape.enum.extrapolation.nearest  R1_vecCell=ModuleType1.R1_vecCell Ohm  tau1_vecCell=ModuleType1.tau1_vecCell s  R2_vecCell=ModuleType1.R2_vecCell Ohm  tau2_vecCell=ModuleType1.tau2_vecCell s  P=1  S=1  iCell_specify=on  iCell_priority=None  iCell=ModuleAssembly6.Module4.iCell A  iCell_nominal_specify=off  iCell_nominal_unit=A  iCell_nominal_value=1  vCell_specify=on  vCell_priority=None  vCell=ModuleAssembly6.Module4.vCell V  vCell_nominal_specify=off  vCell_nominal_unit=V  vCell_nominal_value=1  socCell_specify=on  socCell_priority=High  socCell=ModuleAssembly6.Module4.socCell  socCell_nominal_specify=off  socCell_nominal_unit=1  socCell_nominal_value=1  numCyclesCell_specify=on  numCyclesCell_priority=High  numCyclesCell=ModuleAssembly6.Module4.numCyclesCell  numCyclesCell_nominal_specify=off  numCyclesCell_nominal_unit=1  numCyclesCell_nominal_value=1  vParallelAssembly_specify=on  vParallelAssembly_priority=None  vParallelAssembly=ModuleAssembly6.Module4.vParallelAssembly V  vParallelAssembly_nominal_specify=off  vParallelAssembly_nominal_unit=V  vParallelAssembly_nominal_value=1  socParallelAssembly_specify=on  socParallelAssembly_priority=None  socParallelAssembly=ModuleAssembly6.Module4.socParallelAssembly  socParallelAssembly_nominal_specify=off  socParallelAssembly_nominal_unit=1  socParallelAssembly_nominal_value=1
      settings: InternalSimscapePortConfiguration="{\"Bottom\":[{\"id\":\"n\",\"label\":\"-\",\"type\":\"foundation.electrical.electrical\"}],\"Left\":[],\"Right\":[],\"Top\":[{\"id\":\"p\",\"label\":\"+\",\"type\":\"foundation.electrical.electrical\"}]}"
  Module4_outputs : SimscapeProbe  BoundBlock=3303  Variables={iCell, numCyclesCell, socCell, socParallelAssembly, vCell, vParallelAssembly}
  Module5 : batteryModelFromBlockDetailed2RC_IC_lib/Modules/ModuleType1  SOC_vecCell=ModuleType1.SOC_vecCell  V0_vecCell=ModuleType1.V0_vecCell V  V_rangeCell=ModuleType1.V_rangeCell V  R0_vecCell=ModuleType1.R0_vecCell Ohm  AHCell=ModuleType1.AHCell A*hr  extrapolation_optionCell=simscape.enum.extrapolation.nearest  R1_vecCell=ModuleType1.R1_vecCell Ohm  tau1_vecCell=ModuleType1.tau1_vecCell s  R2_vecCell=ModuleType1.R2_vecCell Ohm  tau2_vecCell=ModuleType1.tau2_vecCell s  P=1  S=1  iCell_specify=on  iCell_priority=None  iCell=ModuleAssembly6.Module5.iCell A  iCell_nominal_specify=off  iCell_nominal_unit=A  iCell_nominal_value=1  vCell_specify=on  vCell_priority=None  vCell=ModuleAssembly6.Module5.vCell V  vCell_nominal_specify=off  vCell_nominal_unit=V  vCell_nominal_value=1  socCell_specify=on  socCell_priority=High  socCell=ModuleAssembly6.Module5.socCell  socCell_nominal_specify=off  socCell_nominal_unit=1  socCell_nominal_value=1  numCyclesCell_specify=on  numCyclesCell_priority=High  numCyclesCell=ModuleAssembly6.Module5.numCyclesCell  numCyclesCell_nominal_specify=off  numCyclesCell_nominal_unit=1  numCyclesCell_nominal_value=1  vParallelAssembly_specify=on  vParallelAssembly_priority=None  vParallelAssembly=ModuleAssembly6.Module5.vParallelAssembly V  vParallelAssembly_nominal_specify=off  vParallelAssembly_nominal_unit=V  vParallelAssembly_nominal_value=1  socParallelAssembly_specify=on  socParallelAssembly_priority=None  socParallelAssembly=ModuleAssembly6.Module5.socParallelAssembly  socParallelAssembly_nominal_specify=off  socParallelAssembly_nominal_unit=1  socParallelAssembly_nominal_value=1
      settings: InternalSimscapePortConfiguration="{\"Bottom\":[{\"id\":\"n\",\"label\":\"-\",\"type\":\"foundation.electrical.electrical\"}],\"Left\":[],\"Right\":[],\"Top\":[{\"id\":\"p\",\"label\":\"+\",\"type\":\"foundation.electrical.electrical\"}]}"
  Module5_outputs : SimscapeProbe  BoundBlock=3305  Variables={iCell, numCyclesCell, socCell, socParallelAssembly, vCell, vParallelAssembly}
  Module6 : batteryModelFromBlockDetailed2RC_IC_lib/Modules/ModuleType1  SOC_vecCell=ModuleType1.SOC_vecCell  V0_vecCell=ModuleType1.V0_vecCell V  V_rangeCell=ModuleType1.V_rangeCell V  R0_vecCell=ModuleType1.R0_vecCell Ohm  AHCell=ModuleType1.AHCell A*hr  extrapolation_optionCell=simscape.enum.extrapolation.nearest  R1_vecCell=ModuleType1.R1_vecCell Ohm  tau1_vecCell=ModuleType1.tau1_vecCell s  R2_vecCell=ModuleType1.R2_vecCell Ohm  tau2_vecCell=ModuleType1.tau2_vecCell s  P=1  S=1  iCell_specify=on  iCell_priority=None  iCell=ModuleAssembly6.Module6.iCell A  iCell_nominal_specify=off  iCell_nominal_unit=A  iCell_nominal_value=1  vCell_specify=on  vCell_priority=None  vCell=ModuleAssembly6.Module6.vCell V  vCell_nominal_specify=off  vCell_nominal_unit=V  vCell_nominal_value=1  socCell_specify=on  socCell_priority=High  socCell=ModuleAssembly6.Module6.socCell  socCell_nominal_specify=off  socCell_nominal_unit=1  socCell_nominal_value=1  numCyclesCell_specify=on  numCyclesCell_priority=High  numCyclesCell=ModuleAssembly6.Module6.numCyclesCell  numCyclesCell_nominal_specify=off  numCyclesCell_nominal_unit=1  numCyclesCell_nominal_value=1  vParallelAssembly_specify=on  vParallelAssembly_priority=None  vParallelAssembly=ModuleAssembly6.Module6.vParallelAssembly V  vParallelAssembly_nominal_specify=off  vParallelAssembly_nominal_unit=V  vParallelAssembly_nominal_value=1  socParallelAssembly_specify=on  socParallelAssembly_priority=None  socParallelAssembly=ModuleAssembly6.Module6.socParallelAssembly  socParallelAssembly_nominal_specify=off  socParallelAssembly_nominal_unit=1  socParallelAssembly_nominal_value=1
      settings: InternalSimscapePortConfiguration="{\"Bottom\":[{\"id\":\"n\",\"label\":\"-\",\"type\":\"foundation.electrical.electrical\"}],\"Left\":[],\"Right\":[],\"Top\":[{\"id\":\"p\",\"label\":\"+\",\"type\":\"foundation.electrical.electrical\"}]}"
  Module6_outputs : SimscapeProbe  BoundBlock=3307  Variables={iCell, numCyclesCell, socCell, socParallelAssembly, vCell, vParallelAssembly}
  NewModule : batteryModelFromBlockDetailed2RC_IC_lib/Modules/ModuleType1  SOC_vecCell=ModuleType1.SOC_vecCell  V0_vecCell=ModuleType1.V0_vecCell V  V_rangeCell=ModuleType1.V_rangeCell V  R0_vecCell=ModuleType1.R0_vecCell Ohm  AHCell=ModuleType1.AHCell A*hr  extrapolation_optionCell=simscape.enum.extrapolation.nearest  R1_vecCell=ModuleType1.R1_vecCell Ohm  tau1_vecCell=ModuleType1.tau1_vecCell s  R2_vecCell=ModuleType1.R2_vecCell Ohm  tau2_vecCell=ModuleType1.tau2_vecCell s  P=1  S=1  iCell_specify=on  iCell_priority=None  iCell=ModuleAssembly6.NewModule.iCell A  iCell_nominal_specify=off  iCell_nominal_unit=A  iCell_nominal_value=1  vCell_specify=on  vCell_priority=None  vCell=ModuleAssembly6.NewModule.vCell V  vCell_nominal_specify=off  vCell_nominal_unit=V  vCell_nominal_value=1  socCell_specify=on  socCell_priority=High  socCell=ModuleAssembly6.NewModule.socCell  socCell_nominal_specify=off  socCell_nominal_unit=1  socCell_nominal_value=1  numCyclesCell_specify=on  numCyclesCell_priority=High  numCyclesCell=ModuleAssembly6.NewModule.numCyclesCell  numCyclesCell_nominal_specify=off  numCyclesCell_nominal_unit=1  numCyclesCell_nominal_value=1  vParallelAssembly_specify=on  vParallelAssembly_priority=None  vParallelAssembly=ModuleAssembly6.NewModule.vParallelAssembly V  vParallelAssembly_nominal_specify=off  vParallelAssembly_nominal_unit=V  vParallelAssembly_nominal_value=1  socParallelAssembly_specify=on  socParallelAssembly_priority=None  socParallelAssembly=ModuleAssembly6.NewModule.socParallelAssembly  socParallelAssembly_nominal_specify=off  socParallelAssembly_nominal_unit=1  socParallelAssembly_nominal_value=1
      settings: InternalSimscapePortConfiguration="{\"Bottom\":[{\"id\":\"n\",\"label\":\"-\",\"type\":\"foundation.electrical.electrical\"}],\"Left\":[],\"Right\":[],\"Top\":[{\"id\":\"p\",\"label\":\"+\",\"type\":\"foundation.electrical.electrical\"}]}"
  NewModule_outputs : SimscapeProbe  BoundBlock=3309  Variables={iCell, numCyclesCell, socCell, socParallelAssembly, vCell, vParallelAssembly}
  iCellMux : Mux  Inputs=6
  numCyclesCellMux : Mux  Inputs=6
  socCellMux : Mux  Inputs=6
  socParallelAssemblyMux : Mux  Inputs=6
  vCellMux : Mux  Inputs=6
  vParallelAssemblyMux : Mux  Inputs=6
  + : PMIOPort  Side=Left
  - : PMIOPort  Port=2  Side=Right
  iCell : Outport
  numCyclesCell : Outport  Port=2
  socCell : Outport  Port=3
  socParallelAssembly : Outport  Port=4
  vCell : Outport  Port=5
  vParallelAssembly : Outport  Port=6
  wires:
  [vParallelAssembly6] -> vParallelAssemblyMux/6
  Module6_outputs/6 -> [vParallelAssembly6]
  [vCell6] -> vCellMux/6
  Module6_outputs/5 -> [vCell6]
  [socParallelAssembly6] -> socParallelAssemblyMux/6
  Module6_outputs/4 -> [socParallelAssembly6]
  [socCell6] -> socCellMux/6
  Module6_outputs/3 -> [socCell6]
  [numCyclesCell6] -> numCyclesCellMux/6
  Module6_outputs/2 -> [numCyclesCell6]
  [iCell6] -> iCellMux/6
  Module6_outputs/1 -> [iCell6]
  [vParallelAssembly5] -> vParallelAssemblyMux/5
  Module5_outputs/6 -> [vParallelAssembly5]
  [vCell5] -> vCellMux/5
  Module5_outputs/5 -> [vCell5]
  [socParallelAssembly5] -> socParallelAssemblyMux/5
  Module5_outputs/4 -> [socParallelAssembly5]
  [socCell5] -> socCellMux/5
  Module5_outputs/3 -> [socCell5]
  [numCyclesCell5] -> numCyclesCellMux/5
  Module5_outputs/2 -> [numCyclesCell5]
  [iCell5] -> iCellMux/5
  Module5_outputs/1 -> [iCell5]
  [vParallelAssembly4] -> vParallelAssemblyMux/4
  Module4_outputs/6 -> [vParallelAssembly4]
  [vCell4] -> vCellMux/4
  Module4_outputs/5 -> [vCell4]
  [socParallelAssembly4] -> socParallelAssemblyMux/4
  Module4_outputs/4 -> [socParallelAssembly4]
  [socCell4] -> socCellMux/4
  Module4_outputs/3 -> [socCell4]
  [numCyclesCell4] -> numCyclesCellMux/4
  Module4_outputs/2 -> [numCyclesCell4]
  [iCell4] -> iCellMux/4
  Module4_outputs/1 -> [iCell4]
  [vParallelAssembly3] -> vParallelAssemblyMux/3
  Module3_outputs/6 -> [vParallelAssembly3]
  [vCell3] -> vCellMux/3
  Module3_outputs/5 -> [vCell3]
  [socParallelAssembly3] -> socParallelAssemblyMux/3
  Module3_outputs/4 -> [socParallelAssembly3]
  [socCell3] -> socCellMux/3
  Module3_outputs/3 -> [socCell3]
  [numCyclesCell3] -> numCyclesCellMux/3
  Module3_outputs/2 -> [numCyclesCell3]
  [iCell3] -> iCellMux/3
  Module3_outputs/1 -> [iCell3]
  [vParallelAssembly2] -> vParallelAssemblyMux/2
  Module2_outputs/6 -> [vParallelAssembly2]
  [vCell2] -> vCellMux/2
  Module2_outputs/5 -> [vCell2]
  [socParallelAssembly2] -> socParallelAssemblyMux/2
  Module2_outputs/4 -> [socParallelAssembly2]
  [socCell2] -> socCellMux/2
  Module2_outputs/3 -> [socCell2]
  [numCyclesCell2] -> numCyclesCellMux/2
  Module2_outputs/2 -> [numCyclesCell2]
  [iCell2] -> iCellMux/2
  Module2_outputs/1 -> [iCell2]
  [vParallelAssembly1] -> vParallelAssemblyMux/1
  vParallelAssemblyMux/1 -> vParallelAssembly/1
  NewModule_outputs/6 -> [vParallelAssembly1]
  [vCell1] -> vCellMux/1
  vCellMux/1 -> vCell/1
  NewModule_outputs/5 -> [vCell1]
  [socParallelAssembly1] -> socParallelAssemblyMux/1
  socParallelAssemblyMux/1 -> socParallelAssembly/1
  NewModule_outputs/4 -> [socParallelAssembly1]
  [socCell1] -> socCellMux/1
  socCellMux/1 -> socCell/1
  NewModule_outputs/3 -> [socCell1]
  [numCyclesCell1] -> numCyclesCellMux/1
  numCyclesCellMux/1 -> numCyclesCell/1
  NewModule_outputs/2 -> [numCyclesCell1]
  [iCell1] -> iCellMux/1
  iCellMux/1 -> iCell/1
  NewModule_outputs/1 -> [iCell1]
  connections:
  Module6/RConn1 -- -/RConn1
  NewModule/LConn1 -- +/RConn1
  Module6/LConn1 -- Module5/RConn1
  Module5/LConn1 -- Module4/RConn1
  Module4/LConn1 -- Module3/RConn1
  Module3/LConn1 -- Module2/RConn1
  Module2/LConn1 -- NewModule/RConn1
